simulink model "suspension_model"  (R2020b)
settings: Solver=VariableStepAuto  StartTime=0.0  StopTime=10  RelTol=1e-3
undefined symbols (not defined in the file or in its folder): B, K1, K2, M1, M2
settings Model: Creator=153  LastModifiedBy=153
settings DataIOCC: ExternalInput=[signal]  LoadExternalInput=on  SaveFormat=Array  SignalLogging=off  DSMLogging=off
settings DebuggingCC: MaxConsecutiveZCsMsg=none  ModelReferenceExtraNoncontSigs=none

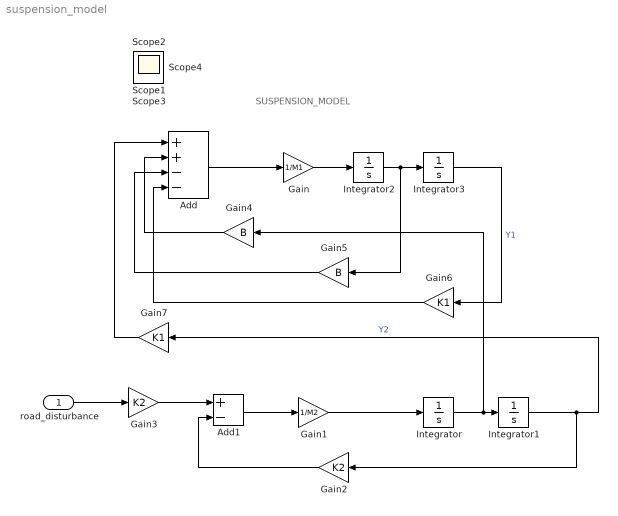
== system suspension_model ==
  note: SUSPENSION_MODEL
  road_disturbance : Inport
  Add : Sum  Inputs=++--
  Add1 : Sum  Inputs=+-
  Gain : Gain  Gain=1/M1
  Gain1 : Gain  Gain=1/M2
  Gain2 : Gain  Gain=K2
  Gain3 : Gain  Gain=K2
  Gain4 : Gain  Gain=B
  Gain5 : Gain  Gain=B
  Gain6 : Gain  Gain=K1
  Gain7 : Gain  Gain=K1
  Integrator{,1..3} (4 alike) : Integrator
  Scope{1..4} (4 alike) : Scope
  wires:
  Gain2/1 -> Add1/2
  Add1/1 -> Gain1/1
  Gain1/1 -> Integrator/1
  Integrator/1 -> Integrator1/1, Gain4/1
  Add/1 -> Gain/1
  Gain/1 -> Integrator2/1
  Integrator2/1 -> Integrator3/1, Gain5/1
  Gain7/1 -> Add/1
  Gain6/1 -> Add/4
  Gain5/1 -> Add/3
  Gain4/1 -> Add/2
  Integrator3/1 -> Gain6/1  "Y1"
  road_disturbance/1 -> Gain3/1
  Gain3/1 -> Add1/1
  Integrator1/1 -> Gain2/1, Gain7/1  "Y2"
